simulink model "Enabled_Subsystem"  (R2021a)
settings: Solver=FixedStepAuto  StartTime=0.0  StopTime=10.0  FixedStep=1e-3  RelTol=1e-3
settings Model: Creator=lenovo  LastModifiedBy=lenovo

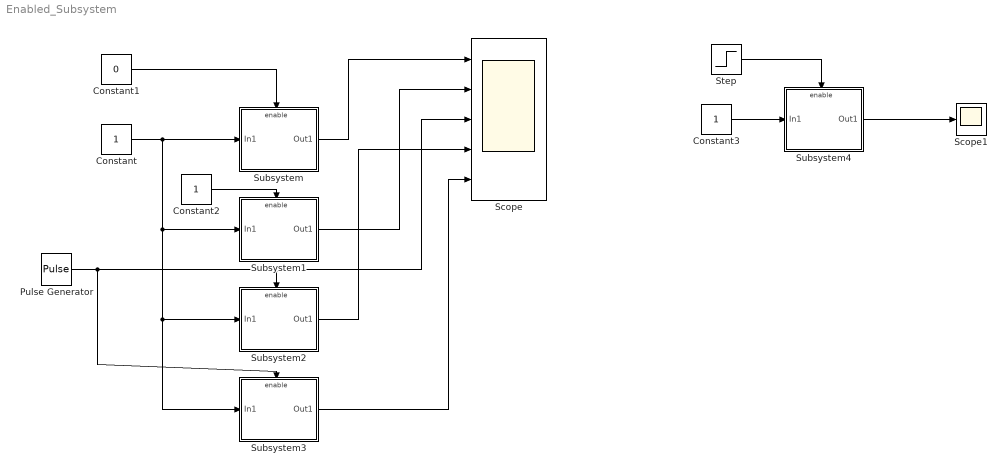
== system Enabled_Subsystem ==
  Constant : Constant
  Constant1 : Constant  Value=0
  Constant2 : Constant
  Constant3 : Constant
  Pulse Generator : DiscretePulseGenerator  PulseType=Time based  PulseWidth=50
  Scope : Scope  NumInputPorts=5
  Scope1 : Scope
  Step : Step  SampleTime=0
  Subsystem : Subsystem
  Subsystem1 : Subsystem
  Subsystem2 : Subsystem
  Subsystem3 : Subsystem
  Subsystem4 : Subsystem
  wires:
  Constant/1 -> Subsystem3/1(In1), Subsystem2/1(In1), Subsystem1/1(In1), Subsystem/1(In1)
  Constant2/1 -> Subsystem1/Enable
  Constant1/1 -> Subsystem/Enable
  Subsystem/1(Out1) -> Scope/1
  Subsystem1/1(Out1) -> Scope/2
  Subsystem2/1(Out1) -> Scope/4
  Subsystem3/1(Out1) -> Scope/5
  Pulse Generator/1 -> Subsystem3/Enable, Scope/3, Subsystem2/Enable
  Constant3/1 -> Subsystem4/1(In1)
  Subsystem4/1(Out1) -> Scope1/1
  Step/1 -> Subsystem4/Enable

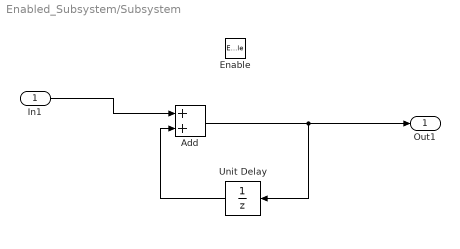
== system Enabled_Subsystem/Subsystem ==
  In1 : Inport
  Enable : EnablePort
  Add : Sum
  Unit Delay : UnitDelay  SampleTime=-1  HasFrameUpgradeWarning=on
  Out1 : Outport
  wires:
  Add/1 -> Out1/1, Unit Delay/1
  Unit Delay/1 -> Add/2
  In1/1 -> Add/1

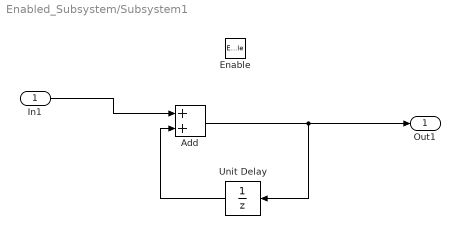
== system Enabled_Subsystem/Subsystem1 ==
  In1 : Inport
  Enable : EnablePort
  Add : Sum
  Unit Delay : UnitDelay  SampleTime=-1  HasFrameUpgradeWarning=on
  Out1 : Outport
  wires:
  In1/1 -> Add/1
  Unit Delay/1 -> Add/2
  Add/1 -> Unit Delay/1, Out1/1

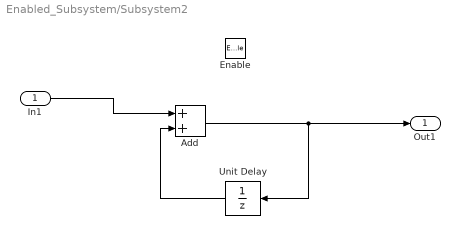
== system Enabled_Subsystem/Subsystem2 ==
  In1 : Inport
  Enable : EnablePort
  Add : Sum
  Unit Delay : UnitDelay  SampleTime=-1  HasFrameUpgradeWarning=on
  Out1 : Outport
  wires:
  Add/1 -> Out1/1, Unit Delay/1
  Unit Delay/1 -> Add/2
  In1/1 -> Add/1

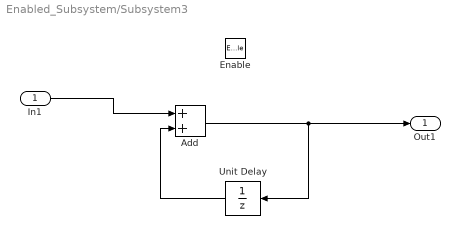
== system Enabled_Subsystem/Subsystem3 ==
  In1 : Inport
  Enable : EnablePort  StatesWhenEnabling=reset
  Add : Sum
  Unit Delay : UnitDelay  SampleTime=-1  HasFrameUpgradeWarning=on
  Out1 : Outport
  wires:
  In1/1 -> Add/1
  Unit Delay/1 -> Add/2
  Add/1 -> Unit Delay/1, Out1/1

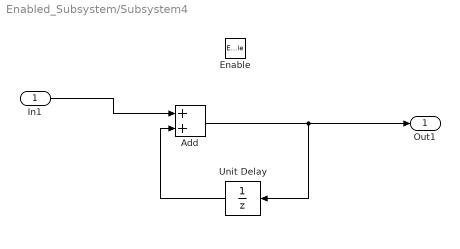
== system Enabled_Subsystem/Subsystem4 ==
  In1 : Inport
  Enable : EnablePort
  Add : Sum
  Unit Delay : UnitDelay  SampleTime=-1  HasFrameUpgradeWarning=on
  Out1 : Outport
  wires:
  In1/1 -> Add/1
  Unit Delay/1 -> Add/2
  Add/1 -> Unit Delay/1, Out1/1
